simulink model "p5p5e_sim"  (Simulink 9.2)
settings: Solver=ode45  StartTime=0.0  StopTime=400  RelTol=1e-3  EnableMultiTasking=on
values from neighbouring files (symbols this model uses):
  T_s = 1/f_s    (= 0.1)    [p5p5c.m]
undefined symbols (not defined in the file or in its folder): psi_r
libraries: simulink_extras x6, simulink x2, cstblocks x2
settings Model: Creator=markh  LastModifiedBy=halvo
settings DataIOCC: SignalLoggingName=sigsOut
settings OptimizationCC: InitFltsAndDblsToZero=on
settings DebuggingCC: SaveWithParameterizedLinksMsg=none  SignalResolutionControl=TryResolveAllWithWarning  MultiTaskDSMMsg=warning  MultiTaskCondExecSysMsg=none
settings HardwareCC: TargetBitPerPointer=64  TargetBitPerSizeT=64  TargetBitPerPtrDiffT=64  TargetLongLongMode=on  TargetIntDivRoundTo=Zero  TargetEndianess=LittleEndian  TargetWordSize=64  TargetHWDeviceType=MATLAB Host  ProdEqTarget=off
settings GRTTargetCC: TargetFcnLib=ansi_tfl_tmw.mat

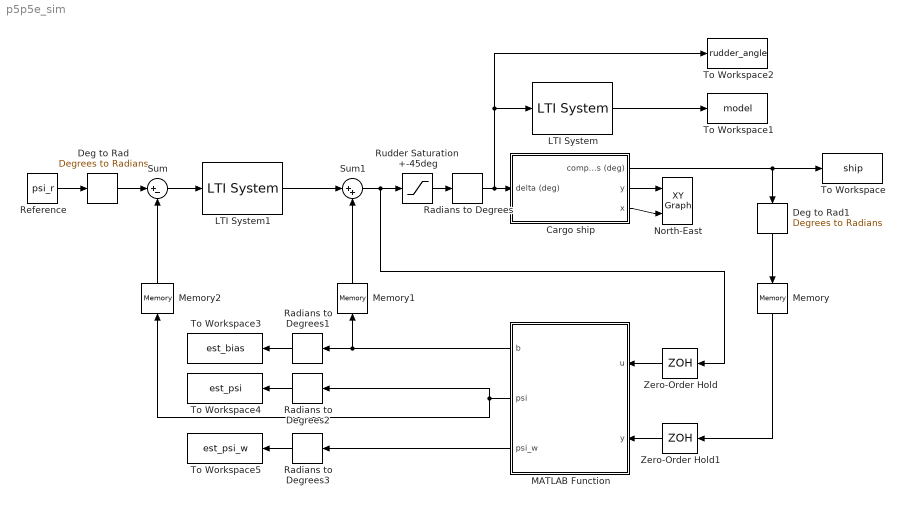
== system p5p5e_sim ==
  Cargo ship : Subsystem  mask(Simple shipmodel for a cargo ship){noise=on, current=on, logic=on}
      mask prompts: noise "measurement noise"; logic "waves"
      mask help:
      | Measurement noise:
      | 	checked = noise on
      | 	unchecked = noise off
      |
      | Current:
      | 	checked = current on
      | 	unchecked = current off
      |
      | Waves:
      | 	checked = waves on
      | 	unchecked = waves off
      |
      | Author: Jørgen Spjøtvold, 9/10-2003
      | TTK 4115 Linear system theory.
      | Modified by Jostein Bakkeheim 26/10-2006
  Deg to Rad : simulink_extras/Transformations/Degrees to Radians
  Deg to Rad1 : simulink_extras/Transformations/Degrees to Radians
  LTI System : cstblocks/LTI System  sys=H_ship  IC=[]
  LTI System1 : cstblocks/LTI System  sys=H_pd  IC=[]
  MATLAB Function : MATLAB Function  TreatAsAtomicUnit=on
  Memory : Memory
  Memory1 : Memory
  Memory2 : Memory
  North-East : simulink/Sinks/XY Graph  xmin=-5000  xmax=5000  ymin=-5000  ymax=5000  st=-1
  Radians to Degrees{,1..3} (4 alike) : simulink_extras/Transformations/Radians to Degrees
  Reference : Constant  Value=psi_r
  Rudder Saturation  +-45deg : Saturate  UpperLimit=45*(pi/180)  LowerLimit=-45*(pi/180)
  Sum : Sum  Inputs=|+-
  Sum1 : Sum  Inputs=|++
  To Workspace : ToWorkspace  VariableName=ship  SaveFormat=Structure With Time  SampleTime=-1
  To Workspace1 : ToWorkspace  VariableName=model  SaveFormat=Structure With Time  SampleTime=-1
  To Workspace2 : ToWorkspace  VariableName=rudder_angle  SaveFormat=Structure With Time  SampleTime=-1
  To Workspace3 : ToWorkspace  VariableName=est_bias  SaveFormat=Structure With Time  SampleTime=-1
  To Workspace4 : ToWorkspace  VariableName=est_psi  SaveFormat=Structure With Time  SampleTime=-1
  To Workspace5 : ToWorkspace  VariableName=est_psi_w  SaveFormat=Structure With Time  SampleTime=-1
  Zero-Order Hold : ZeroOrderHold  SampleTime=T_s
  Zero-Order Hold1 : ZeroOrderHold  SampleTime=T_s
  wires:
  Cargo ship/3(x) -> North-East/2
  Cargo ship/2(y) -> North-East/1
  Reference/1 -> Deg to Rad/1
  Deg to Rad/1 -> Sum/1
  Sum/1 -> LTI System1/1
  LTI System/1 -> To Workspace1/1
  Memory/1 -> Zero-Order Hold1/1
  Zero-Order Hold1/1 -> MATLAB Function/2(y)
  Zero-Order Hold/1 -> MATLAB Function/1(u)
  Sum1/1 -> Rudder Saturation  +-45deg/1, Zero-Order Hold/1
  LTI System1/1 -> Sum1/1
  Cargo ship/1(compass (deg)) -> To Workspace/1, Deg to Rad1/1
  Deg to Rad1/1 -> Memory/1
  MATLAB Function/1(b) -> Radians to Degrees1/1, Memory1/1
  Radians to Degrees1/1 -> To Workspace3/1
  Radians to Degrees2/1 -> To Workspace4/1
  MATLAB Function/2(psi) -> Radians to Degrees2/1, Memory2/1
  MATLAB Function/3(psi_w) -> Radians to Degrees3/1
  Radians to Degrees3/1 -> To Workspace5/1
  Radians to Degrees/1 -> To Workspace2/1, LTI System/1, Cargo ship/1(delta (deg))
  Rudder Saturation  +-45deg/1 -> Radians to Degrees/1
  Memory1/1 -> Sum1/2
  Memory2/1 -> Sum/2

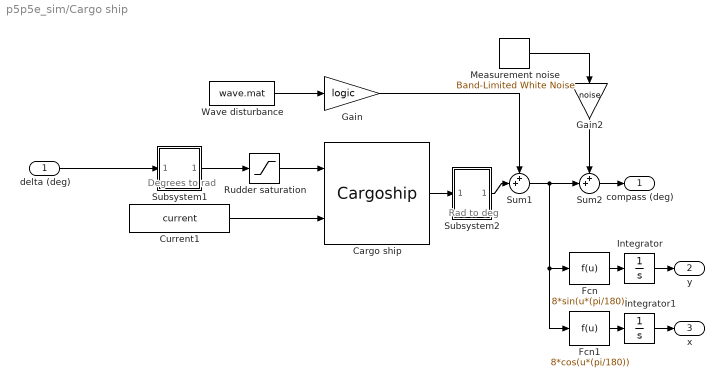
== system p5p5e_sim/Cargo ship ==
  note: Degrees to rad
  note: Rad to deg
  delta (deg) : Inport
  Cargo ship : S-Function  FunctionName=Cargoship  SFunctionDeploymentMode=off  EnableBusSupport=off  mask(Cargo ship){}
      mask help:
      | S-function which simulates a cargo ship.
      |
      | Author: Jørgen Spjøtvold
      | 20.10-2003
      | Modified by Jostein Bakkeheim 27.10.2006
  Current1 : Constant  Value=current
  Fcn : Fcn  Expr=8*sin(u*(pi/180))
  Fcn1 : Fcn  Expr=8*cos(u*(pi/180))
  Gain : Gain  Gain=logic  SaturateOnIntegerOverflow=on  OutDataTypeStr=Inherit: Same as input  ParamDataTypeStr=Inherit: Same as input
  Gain2 : Gain  Gain=noise  SaturateOnIntegerOverflow=on  OutDataTypeStr=Inherit: Same as input  ParamDataTypeStr=Inherit: Same as input
  Integrator : Integrator
  Integrator1 : Integrator
  Measurement noise : simulink/Sources/Band-Limited White Noise  Cov=[0.001]  Ts=.5  seed=[23341]
  Rudder saturation : Saturate  UpperLimit=45*(pi/180)  LowerLimit=-45*(pi/180)
  Subsystem1 : Subsystem  mask(degrees to radians){}
      mask help: Converts degrees to radians
      mask Display: fprintf('D2R');
  Subsystem2 : Subsystem  mask(radians to degrees){}
      mask help: Converts radians to degrees
      mask Display: fprintf('R2D');
  Sum1 : Sum  Inputs=++|  SaturateOnIntegerOverflow=on
  Sum2 : Sum  Inputs=++|  SaturateOnIntegerOverflow=on
  Wave disturbance : FromFile  FileName=wave.mat  SampleTime=0
  compass (deg) : Outport
  y : Outport  Port=2
  x : Outport  Port=3
  wires:
  delta (deg)/1 -> Subsystem1/1(In1)
  Fcn/1 -> Integrator/1
  Integrator/1 -> y/1
  Fcn1/1 -> Integrator1/1
  Integrator1/1 -> x/1
  Wave disturbance/1 -> Gain/1
  Subsystem2/1(Out1) -> Sum1/2
  Gain/1 -> Sum1/1
  Sum1/1 -> Fcn/1, Fcn1/1, Sum2/2
  Cargo ship/1 -> Subsystem2/1(In1)
  Subsystem1/1(Out1) -> Rudder saturation/1
  Rudder saturation/1 -> Cargo ship/1
  Sum2/1 -> compass (deg)/1
  Measurement noise/1 -> Gain2/1
  Gain2/1 -> Sum2/1
  Current1/1 -> Cargo ship/2

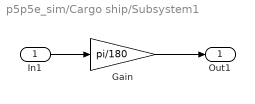
== system p5p5e_sim/Cargo ship/Subsystem1 ==
  In1 : Inport
  Gain : Gain  Gain=pi/180  SaturateOnIntegerOverflow=on  OutDataTypeStr=Inherit: Same as input  ParamDataTypeStr=Inherit: Same as input
  Out1 : Outport
  wires:
  Gain/1 -> Out1/1
  In1/1 -> Gain/1

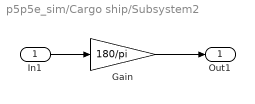
== system p5p5e_sim/Cargo ship/Subsystem2 ==
  In1 : Inport
  Gain : Gain  Gain=180/pi  SaturateOnIntegerOverflow=on  OutDataTypeStr=Inherit: Same as input  ParamDataTypeStr=Inherit: Same as input
  Out1 : Outport
  wires:
  Gain/1 -> Out1/1
  In1/1 -> Gain/1

== matlab function MATLAB Function ==
  data: u input double; b output double; y input double; psi output double; psi_w output double
function [b, psi, psi_w] = kalman_filter_func(u, y)
    persistent init_flag A B C E Q R_v P_ x_ I

    if isempty(init_flag)
        init_flag = 1;
        
        %initialize the matrices
        
        matrices = load('task_55.mat');
        A = matrices.A_d;
        B = matrices.B_d;
        C = matrices.C_d;
        E = matrices.E_d;
        Q = matrices.Q;
        R_v = matrices.R_v;
        P_ = matrices.P_;
        x_ = matrices.x_;
        I = matrices.I;
    end
    
    %update with measurement
    K = P_*C'*inv(C*P_*C' + R_v);         %Kalman gain
    x = x_ + K*(y-C*x_);                  %Linear observer
    P = (I-K*C)*P_*(I-K*C)' + K*R_v*K'; %Update error covariance
    
    %predict for next step
    x_ = A*x + B*u;
    P_ = A*P*A' + E*Q*E';
    
    b = x(5);
    psi = x(3);
    psi_w = x(2);
end
